simulink model "simDCmotorFLC"  (R2018a)
settings: Solver=VariableStepAuto  StartTime=0.0  StopTime=30  RelTol=1e-3
libraries: fuzblock x1
settings Model: Creator=Teo  LastModifiedBy=Teo

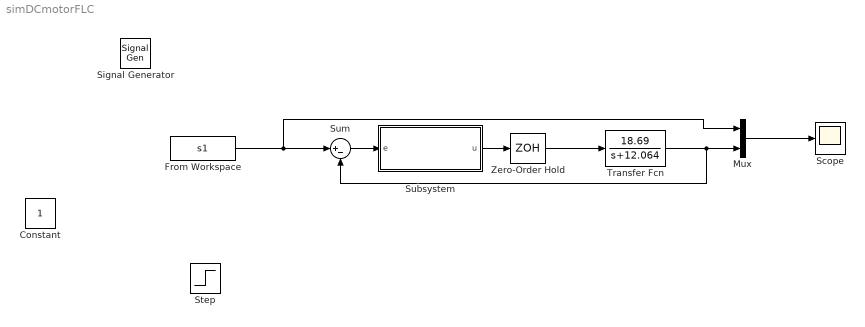
== system simDCmotorFLC ==
  Constant : Constant
  From Workspace : FromWorkspace  VariableName=s1  SampleTime=0.01
  Mux : Mux  Inputs=2
  Scope : Scope
  Signal Generator : SignalGenerator  Units=rad/sec
  Step : Step  Time=10  Before=150  After=150  SampleTime=0
  Subsystem : Subsystem
  Sum : Sum  Inputs=|+-
  Transfer Fcn : TransferFcn  Numerator=[18.69]  Denominator=[1 12.064]
  Zero-Order Hold : ZeroOrderHold  SampleTime=0.01
  wires:
  Zero-Order Hold/1 -> Transfer Fcn/1
  Sum/1 -> Subsystem/1("e ")
  Subsystem/1(u) -> Zero-Order Hold/1
  Mux/1 -> Scope/1
  Transfer Fcn/1 -> Sum/2, Mux/2
  From Workspace/1 -> Sum/1, Mux/1

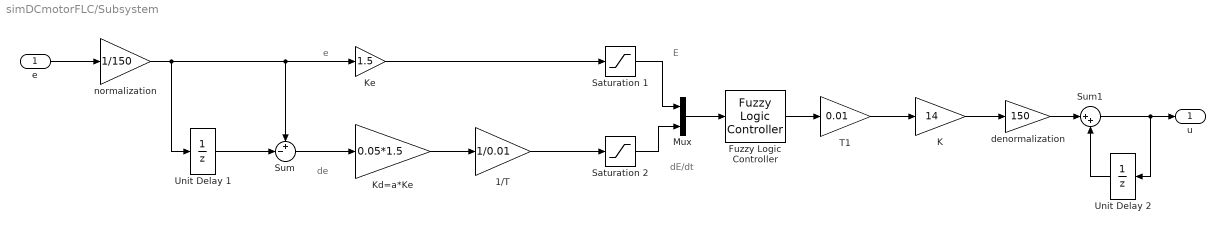
== system simDCmotorFLC/Subsystem ==
  note: e
  note: E
  note: dE/dt
  note: de
  "e " : Inport
  1/T : Gain  Gain=1/0.01  SaturateOnIntegerOverflow=on  OutDataTypeStr=Inherit: Same as input  ParamDataTypeStr=Inherit: Same as input
  Fuzzy Logic Controller : fuzblock/Fuzzy Logic  Controller  FIS=dcmotor  OutputSampleNumber=101  DataType=double  FuzzifiedInputs=off  RuleFiringStrengths=off  RuleOutputs=off  AggregatedOutputs=off  SimulateUsing=Interpreted execution  OutOfRangeInputValueMessage=warning  NoRuleFiredMessage=warning  EmptyOutputFuzzySetMessage=warning
  K : Gain  Gain=14  SaturateOnIntegerOverflow=on  OutDataTypeStr=Inherit: Same as input  ParamDataTypeStr=Inherit: Same as input
  Kd=a*Ke : Gain  Gain=0.05*1.5  SaturateOnIntegerOverflow=on  OutDataTypeStr=Inherit: Same as input  ParamDataTypeStr=Inherit: Same as input
  Ke : Gain  Gain=1.5  SaturateOnIntegerOverflow=on
  Mux : Mux  Inputs=2
  Saturation 1 : Saturate  UpperLimit=1  LowerLimit=-1
  Saturation 2 : Saturate  UpperLimit=1  LowerLimit=-1
  Sum : Sum  Inputs=+-|
  Sum1 : Sum  Inputs=|++  SaturateOnIntegerOverflow=on
  T1 : Gain  Gain=0.01  SaturateOnIntegerOverflow=on  OutDataTypeStr=Inherit: Same as input  ParamDataTypeStr=Inherit: Same as input
  Unit Delay 1 : UnitDelay  SampleTime=0.01
  Unit Delay 2 : UnitDelay  SampleTime=0.01
  denormalization : Gain  Gain=150  SaturateOnIntegerOverflow=on  OutDataTypeStr=Inherit: Same as input  ParamDataTypeStr=Inherit: Same as input
  normalization : Gain  Gain=1/150  SaturateOnIntegerOverflow=on  OutDataTypeStr=Inherit: Same as input  ParamDataTypeStr=Inherit: Same as input
  u : Outport
  wires:
  Unit Delay 1/1 -> Sum/2
  Sum/1 -> Kd=a*Ke/1
  Unit Delay 2/1 -> Sum1/2
  Sum1/1 -> u/1, Unit Delay 2/1
  denormalization/1 -> Sum1/1
  K/1 -> denormalization/1
  T1/1 -> K/1
  Saturation 2/1 -> Mux/2
  Saturation 1/1 -> Mux/1
  1/T/1 -> Saturation 2/1
  Kd=a*Ke/1 -> 1/T/1
  Ke/1 -> Saturation 1/1
  Mux/1 -> Fuzzy Logic Controller/1
  Fuzzy Logic Controller/1 -> T1/1
  "e "/1 -> normalization/1
  normalization/1 -> Unit Delay 1/1, Ke/1, Sum/1
